simulink model "cart"  (R2016a)
settings: Solver=ode45  StartTime=0.0  StopTime=100  MaxStep=.1  RelTol=1e-3
model workspace (MAT data in the model file):
  c = 0.05
  k = 1
  m = 1
settings Model: Creator=emiller  LastModifiedBy=emiller
settings GRTTargetCC: GeneratePreprocessorConditionals=Use local settings

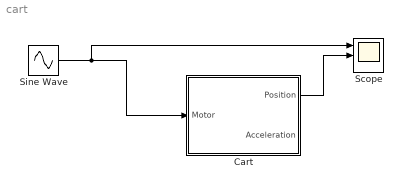
== system cart ==
  Cart : Subsystem
  Scope : Scope  NumInputPorts=3
  Sine Wave : Sin  Amplitude=.02  Frequency=1.39  SampleTime=0
  wires:
  Cart/1(Position) -> Scope/2
  Sine Wave/1 -> Scope/1, Cart/1(Motor)

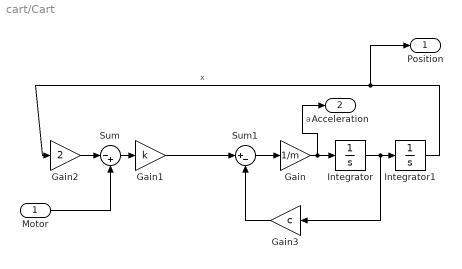
== system cart/Cart ==
  Motor : Inport
  Gain : Gain  Gain=1/m
  Gain1 : Gain  Gain=k
  Gain2 : Gain  Gain=2
  Gain3 : Gain  Gain=c
  Integrator : Integrator
  Integrator1 : Integrator
  Sum : Sum  Inputs=|-+
  Sum1 : Sum  Inputs=|+-
  Position : Outport
  Acceleration : Outport  Port=2
  wires:
  Gain3/1 -> Sum1/2
  Gain1/1 -> Sum1/1
  Sum/1 -> Gain1/1
  Gain2/1 -> Sum/1
  Gain/1 -> Acceleration/1, Integrator/1  "a"
  Integrator/1 -> Gain3/1, Integrator1/1
  Motor/1 -> Sum/2
  Integrator1/1 -> Gain2/1, Position/1  "x"
  Sum1/1 -> Gain/1
